simulink library "DAMA_lib"  (Simulink 6.6)
undefined symbols (not defined in the file or in its folder): aa2rot, D, DiscIntNeverNeededParam, DRprogressbar, epsilon, Kd, Ko, Kp, manip, manipulator, path_des, Q, q0, q_d0, rho, robot, show_3D, StartTime, subs, Ts, VR_handle, vrmfunc
libraries: DAMA_lib x7, vrlib x1, simulink x1
(part 1 of 4)
settings Model: Creator=dario  LastModifiedBy=mofo  ExtModeAutoUpdateStatusClock=off

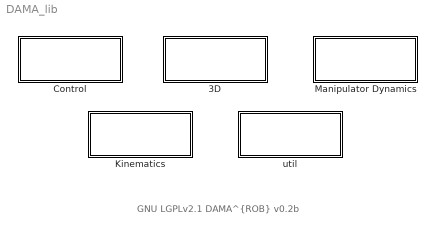
== system DAMA_lib ==
  note: GNU LGPLv2.1 DAMA^{ROB} v0.2b
  3D : Subsystem
  Control : Subsystem
  Kinematics : Subsystem
  Manipulator Dynamics : Subsystem
  util : Subsystem

== system DAMA_lib/3D ==
  note: GNU LGPLv2.1 DAMA^{ROB} v0.2b
  3Dmodel : Subsystem  mask(3D model){sel_obj_nam=Manipulator Name, robot=manipulator, wrlfile=manipVR_base.wrl, SampleTime=0.1, show_ax=off, show_3D_param=off, CaptureFileFormat=png, CaptureFileName='%f_shot_%n.png', Record3D=off, Record3DFileName='%f_anim_%n.wrl', Record2D=off, Record2DCompressMethod=none, Record2DFPS=15, Record2DFileName='%f_anim_%n.avi', Wireframe=off, Viewpoint=STD, RecordMode=scheduled, RecordInterval=[0 10]}
      mask prompts: sel_obj_nam "Input Method"; robot "Manipulator Name"; wrlfile "WRL file name"; SampleTime "3D Sample Time"; show_ax "enable "show axes" input"; show_3D_param "show VRML parameters"; CaptureFileFormat "screenshot file format"; CaptureFileName "screenshot file name (string)"; Record3D "RecordWRL"; Record3DFileName "WRL file name (string)"; Record2D "Record AVI"; Record2DCompressMethod "AVI Compression"; Record2DFPS "AVI FPS"; Record2DFileName "AVI file name (string)"; RecordInterval "Record Interval"
      mask help:
      | Display the 3D model associated with a manipulator.
      |
      | Block Inputs:
      | 1st: signal with joint positions
      | 2nd (if enabled): logical input, if true show frame-axes in 3D animation.
      |
      | Copyright (C) 2009, by Carmine Dario Bellicoso and Marco Caputano.
      | This file is part of DAMA^{ROB} v.???
      | relased under GNU license LGPLv2.1
      mask init:
      | %% SOME INIT
      | mainblock = gcb;
      | blocks = get(gcbh,'Blocks');
      | load_system('DAMA_lib');
      | VR_handle = get_param([gcb,'/VR'],'Handle');
      | % StartTime = str2num(get_param(gcs,'StartTime'));
      | 
      | if strcmp(get_param(gcs,'SimulationStatus'),'stopped')  % operate inside the block only simulation is not running
      |     %% there's something inside the block, delete everything but the inport and VR!
      |     if length(blocks) >= 2
      |         lin = get_param(mainblock,'lines');     % delete lines
      |         if ~isempty(lin)
      |             delete(lin.Handle);
      |         end
      |         for i = 2:1:length(blocks)              % delete blocks
      |             if strcmp(blocks{i},'VR') ~= 1
      |                 delete_block([mainblock,'/',blocks{i}])
      |             end
      |         end
      |         set_param(mainblock,'MaskDisplay', 'disp(''select manipulator'')' );    % change mask aspect
      |         orig_pos = get_param(mainblock,'Position');
      |         new_pos = orig_pos([1,2,1,2]) + [ 0 0 170 65];
      |         set_param(mainblock,'Position', new_pos);
      |     end
      | 
      | 
      |     %% extract information from input data (oject name / WRL file)
      |     if strcmp(sel_obj_nam,'Manipulator Name')
      |         if isa( robot, 'manipulator') && (robot.DH.r ~= 0)
      |             robot_name = robot.name;
      |             DH = robot.DH.table;
      |             r = size(DH)*[1;0];
      |             wrlfile = [robot_name,'VR_base.wrl'];
      |             imagefile = [robot_name,'_3D.png'];
      |         else
      |             return
      |         end
      |     else
      |         if strcmp(sel_obj_nam,'WRL file name')           % WRL file
      |             if exist(wrlfile,'file')
      |                 robot_name = wrlfile(1:end-11);
      |                 imagefile = [robot_name,'_3D.png'];
      |                 f = fopen(wrlfile,'r');
      |                 DH5 = fgetl(f);  %#ok<NASGU>
      |                 DH5 = fgetl(f);
      |                 DH5 = DH5(11:end);
      |                 fclose(f);
      |                 DH5n = eval(DH5);
      |                 r = length(DH5n);
      |                 DH(:,5) = DH5n;
      |             else
      |                 return
      |             end
      |         end
      |     end
      | 
      |     %% specified manipulator or WRL file exists, let's create the subsystem!
      |     if ~exist(imagefile,'file')
      |         imagefile = 'dama_150.png';
      |     end
      |     png = imread(imagefile);
      |     dimY_png = size(png)*[1; 0; 0];
      |     dimX_png = size(png)*[0; 1; 0];
      |     if dimY_png >= 150
      |         dimY = 150;
      |         dimX = round(dimY * dimX_png/dimY_png);
      |     else
      |         dimY = dimY_png;
      |         dimX = dimX_png;
      |     end
      |     Mask_Disp_string = ['image(imread(''',imagefile,'''))',';port_label(''input'',1,''q'');'];
      |     nodes = '';         % VRML nodes to modify
      |     for i = 1:1:r
      |         if DH(i,5) == 0
      |             nodes = [nodes, 'Z', num2str(i-1) ,'.rotation.4.1.double#' ];  %#ok<AGROW>
      |         else
      |             nodes = [nodes, 'Link',num2str(i),'.translation.3#' ];  %#ok<AGROW>
      |         end
      |     end
      | 
      |     for i = 1:1:r
      |         nodes = [nodes,'Xaxis',num2str(i-1),'.scale#']; %#ok<AGROW>
      |         nodes = [nodes,'Yaxis',num2str(i-1),'.scale#']; %#ok<AGROW>
      |         nodes = [nodes,'Zaxis',num2str(i-1),'.scale#']; %#ok<AGROW>
      |     end
      |     nodes = nodes(1:end-1);
      | 
      |     % add demux and connect input 'q' to it
      |     add_block('built-in/demux', [mainblock,'/demux'],...
      |         'DisplayOption','bar',...
      |         'Position','[90,29,95,211]',...
      |         'ShowName','off',...
      |         'Outputs',num2str(r));
      |     add_line(mainblock,'q/1','demux/1');
      | 
      |     % modify VR sink
      |     set_param([mainblock,'/VR'],...
      |         'Position','[360,69,455,141]',...
      |         'WorldFileName',wrlfile,...
      |         'WorldDescription',['3DAMA manipulator: ',robot_name],...
      |         'AutoView','off',...
      |         'SampleTime',num2str(SampleTime),...
      |         'FieldsWritten',nodes, ...
      |         'FigureProperties', '{''Position'', ''Name'', ''Viewpoint'', ''CameraBound'', ''CameraDirection'', ''CameraPosition'', ''CameraUpVector'', ''ZoomFactor'', ''Antialiasing'', ''Headlight'', ''Lighting'', ''NavPanel'', ''StatusBar'', ''ToolBar'', ''Textures'', ''Transparency'', ''Wireframe'', ''NavZones'', ''NavMode'', ''NavSpeed'', ''Record2DCompressMethod'', ''Record2DCompressQuality'', ''Record2D'', ''Record2DFileName'', ''Record2DFPS'';                [5.0000000000000000e+00   9.7000000000000000e+01   7.8400000000000000e+02   5.3800000000000000e+02], ''scara'', ''_untitled_1'', ''on'', [-1.9898756659875949e-02   1.7901367086524811e-01  -9.8364533503023699e-01], [8.8076866149981403e-01  -7.9236092358681276e+00  -7.2561079645852544e-01], [1.9965352243806467e-03   9.8384528836631602e-01   1.7900967126522893e-01], [1.0000000000000000e+00], ''on'', ''on'', ''on'', ''halfbar'', ''on'', ''on'', ''on'', ''on'', ''off'', ''off'', ''examine'', ''normal'', ''auto'', [7.5000000000000000e+01], ''on'', ''%f_anim2_%n.avi'', [1.0000000000000000e+01]}' );
      | 
      |     % add VR rotation and VR translation blocks, with offset and connections
      |     for i = 1:1:length( DH(:,5) )
      |         position = [200, 50, 270, 80] + [0 50 0 50]*(i-1);
      |         if DH(i,5) == 0
      |             add_block('DAMA_lib/util/rotation', [mainblock,'/rotation',num2str(i)]);
      |             set_param([mainblock,'/rotation',num2str(i)],'Position',position);
      |             add_block('built-in/constant', [mainblock,'/offset',num2str(i)]);
      |             set_param([mainblock,'/offset',num2str(i)],'Value','0');                                         % OFFSET HERE
      |             set_param([mainblock,'/offset',num2str(i)],'Position',position - [65,-18,95,-2]);
      |             add_line(mainblock,['rotation',num2str(i),'/1'], ['VR/',num2str(i)]);
      |             add_line(mainblock,['offset',num2str(i),'/1'],['rotation',num2str(i),'/2']);
      |             add_line(mainblock,['demux/',num2str(i)],['rotation',num2str(i),'/1']);
      |         else
      |             add_block('DAMA_lib/util/translation', [mainblock,'/translation',num2str(i)]);
      |             set_param([mainblock,'/translation',num2str(i)],'Position',position);
      |             add_block('built-in/constant', [mainblock,'/offset',num2str(i)]);
      |             set_param([mainblock,'/offset',num2str(i)],'Value','0.5');                                         % OFFSET HERE
      |             set_param([mainblock,'/offset',num2str(i)],'Position',position - [65,-18,95,-2]);
      |             add_line(mainblock,['translation',num2str(i),'/1'], ['VR/',num2str(i)]);
      |             add_line(mainblock,['offset',num2str(i),'/1'],['translation',num2str(i),'/2']);
      |             add_line(mainblock,['demux/',num2str(i)],['translation',num2str(i),'/1']);
      |         end
      |     end
      | 
      |     % add scale control for axes
      |     add_block('built-in/Product',[mainblock,'/show'],...
      |         'Position',[435,212,475,248]);
      |     add_block('built-in/Constant',[mainblock,'/scale'],...
      |         'Value','[1,1,1]',...
      |         'Position','[370,232,410,248]');
      |     add_line(mainblock,'scale/1','show/2');
      |     for i=r+1:1:r+(3*r)
      |         add_line(mainblock,'show/1',['VR/',num2str(i)]);
      |     end
      | 
      |     % inport 2 or constant '1'
      |     if strcmp(get_param(mainblock,'show_ax'),'on')
      |         add_block('built-in/Inport',[mainblock,'/axes_en'],...
      |             'Position','[375,203,405,217]');
      |         Mask_Disp_string = [Mask_Disp_string ,';port_label(''input'',2,''axes'');'];
      |     else
      |         add_block('built-in/Constant',[mainblock,'/axes_en'],...
      |             'Value','1',...
      |             'Position','[375,203,405,217]');
      |     end
      |     add_line(mainblock,'axes_en/1','show/1');
      | 
      |     % change mask aspect
      |     set_param(mainblock,'MaskDisplay',Mask_Disp_string);
      |     orig_pos = get_param(mainblock,'Position');
      |     new_pos = orig_pos([1,2,1,2]) + [ 0 0 dimX dimY];
      |     set_param(mainblock,'Position', new_pos);
      | 
      |     % add 'show 3D' block
      |     %     add_block('DAMA_lib/util/show_3D', [mainblock,'/Show_3D'], ...
      |     %         'Position','[375,286,448,316]');
      | 
      |     vrmfunc('FnOpen', VR_handle );
      |     try
      |         wrl_file = get(get_param([mainblock,'/VR'],'Handle'),'WorldFileName');
      |         list_world_corresp = strfind(get(vrworld(vrsfunc('VRT3ListScenes')),'FileName'),wrl_file);
      |         if length(list_world_corresp) == 1
      |             num_world_found = 1;
      |         else
      |             for i=1:length(list_world_corresp)
      |                 if ~isempty(list_world_corresp{i})
      |                     num_world_found = i;
      |                     break
      |                 end
      |             end
      |         end
      |         ls_wrworlds = vrwho;
      | 
      |         w = ls_wrworlds(num_world_found);
      |         f = get(w, 'Figures');
      |     catch
      |         w = vrworld;
      |         f = vrfigure;
      |     end
      | 
      |     if isvalid(w)
      |         if RecordMode == 1
      |             set(w,'RecordMode','manual');
      |         else
      |             set(w,'RecordMode','scheduled');
      |         end
      |         set(w,'RecordInterval', RecordInterval);
      | 
      |         if Record3D == 0
      |             set(w,'Record3D','off');
      |         else
      |             set(w,'Record3D','on');
      |         end
      |         set(w,'Record3DFileName',Record3DFileName);
      |     end
      | 
      |     if isvalid(f)
      |         if CaptureFileFormat == 1
      |             set(f,'CaptureFileFormat','png');
      |         else
      |             set(f,'CaptureFileFormat','tif');
      |         end
      | 
      |         if Record2D == 0
      |             set(f,'Record2D','off');
      |         else
      |             set(f,'Record2D','on');
      |         end
      | 
      |         if Record2DCompressMethod == 1
      |             set(f,'Record2DCompressMethod','none');
      |         else
      |             set(f,'Record2DCompressMethod','auto');
      |         end
      | 
      |         if Wireframe == 0
      |             set(f,'Wireframe','off');
      |         else
      |             set(f,'Wireframe','on');
      |         end
      | 
      |         if Viewpoint == 1
      |             set(f,'Viewpoint','STD');
      |         elseif Viewpoint == 2
      |             set(f,'Viewpoint','XY_plane');
      |         elseif Viewpoint == 3
      |             set(f,'Viewpoint','XY_perspective');
      |         elseif Viewpoint == 4
      |             set(f,'Viewpoint','left view (XZ)');
      |         elseif Viewpoint == 5
      |             set(f,'Viewpoint','right view (-XZ)');
      |         elseif Viewpoint == 6
      |             set(f,'Viewpoint','rear view (-YZ)');
      |         elseif Viewpoint == 7
      |             set(f,'Viewpoint','front view (-YZ)');
      |         end
      | 
      |         set(f,'Record2DFPS',Record2DFPS);
      |         set(f,'CaptureFileName',CaptureFileName);
      |         set(f,'Record2DFileName',Record2DFileName);
      |     end
      | 
      | else
      | 
      |     try
      |         wrl_file = get(get_param([mainblock,'/VR'],'Handle'),'WorldFileName');
      |         list_world_corresp = strfind(get(vrworld(vrsfunc('VRT3ListScenes')),'FileName'),wrl_file);
      |         if length(list_world_corresp) == 1
      |             num_world_found = 1;
      |         else
      |             for i=1:length(list_world_corresp)
      |                 if ~isempty(list_world_corresp{i})
      |                     num_world_found = i;
      |                     break
      |                 end
      |             end
      |         end
      |         ls_wrworlds = vrwho;
      | 
      |         w = ls_wrworlds(num_world_found);
      |         f = get(w, 'Figures');
      |         if isempty(f)
      |             vrmfunc('FnOpen', VR_handle );
      |         end
      |     catch
      |         w = vrworld;
      |         f = vrfigure;
      |     end
      | 
      |     if isvalid(w)
      |         if RecordMode == 1
      |             set(w,'RecordMode','manual');
      |         else
      |             set(w,'RecordMode','scheduled');
      |         end
      |         set(w,'RecordInterval', RecordInterval);
      | 
      |         if Record3D == 0
      |             set(w,'Record3D','off');
      |         else
      |             set(w,'Record3D','on');
      |         end
      |         set(w,'Record3DFileName',Record3DFileName);
      |     end
      | 
      |     if isvalid(f)
      |         if CaptureFileFormat == 1
      |             set(f,'CaptureFileFormat','png');
      |         else
      |             set(f,'CaptureFileFormat','tif');
      |         end
      | 
      |         if Record2D == 0
      |             set(f,'Record2D','off');
      |         else
      |             set(f,'Record2D','on');
      |         end
      | 
      |         if Record2DCompressMethod == 1
      |             set(f,'Record2DCompressMethod','none');
      |         else
      |             set(f,'Record2DCompressMethod','auto');
      |         end
      | 
      |         if Wireframe == 0
      |             set(f,'Wireframe','off');
      |         else
      |             set(f,'Wireframe','on');
      |         end
      | 
      |         if Viewpoint == 1
      |             set(f,'Viewpoint','STD');
      |         elseif Viewpoint == 2
      |             set(f,'Viewpoint','XY_plane');
      |         elseif Viewpoint == 3
      |             set(f,'Viewpoint','XY_perspective');
      |         elseif Viewpoint == 4
      |             set(f,'Viewpoint','left view (XZ)');
      |         elseif Viewpoint == 5
      |             set(f,'Viewpoint','right view (-XZ)');
      |         elseif Viewpoint == 6
      |             set(f,'Viewpoint','rear view (-YZ)');
      |         elseif Viewpoint == 7
      |             set(f,'Viewpoint','front view (-YZ)');
      |         end
      | 
      |         set(f,'Record2DFPS',Record2DFPS);
      |         set(f,'CaptureFileName',CaptureFileName);
      |         set(f,'Record2DFileName',Record2DFileName);
      |     end
      | end
      mask StyleString: popup(Manipulator Name|WRL file name),edit,edit,edit,checkbox,checkbox,popup(png|tif),edit,checkbox,edit,checkbox,popup(none|auto),edit,edit,checkbox,popup(STD|XY_plane|XY_perspective|left view (XZ)|right view (-XZ)|rear view (-YZ)|front view (-YZ)),popup(manual|scheduled),edit
      mask CallbackString:
      | maskStr = get_param(gcb,'MaskValues');
      | Mask_Vis_Cell_Param = get_param(gcb,'MaskVisibilities');
      | 
      | if strcmp(maskStr{1},'Manipulator Name')
      |     Mask_Vis_Cell_Param{2} = 'on';
      |     Mask_Vis_Cell_Param{3} = 'off';
      | else
      |     Mask_Vis_Cell_Param{2} = 'off';
      |     Mask_Vis_Cell_Param{3} = 'on';
      | end
      | 
      | set_param(gcb,'MaskVisibilities', Mask_Vis_Cell_Param);
      | clear maskStr Mask_Vis_Cell_Param|if strcmp(get_param(gcb,'sel_obj_nam'),'Manipulator Name')
      |     manip_name_param = get_param(gcb,'robot');
      |     if exist(manip_name_param,'var') && isa( eval(manip_name_param), 'manipulator')
      |         % do nothing
      |     else
      |         warndlg([manip_name_param,' is not a valid manipulator name.'])
      |     end
      | end
      | clear manip_name_param|if strcmp(get_param(gcb,'sel_obj_nam'),'WRL file name')
      |     wrl_file_name_param = get_param(gcb,'wrlfile');
      |     if exist(wrl_file_name_param,'file')
      |         % do nothing
      |     else
      |         warndlg([wrl_file_name_param,' does''nt exist.'])
      |     end
      | end
      | clear wrl_file_name_param|||maskStr = get_param(gcb,'MaskValues');
      | Mask_Vis_Cell_Param = get_param(gcb,'MaskVisibilities');
      | 
      | if strcmp(maskStr{6},'on')
      |     for i_mask_par=7:18
      |         Mask_Vis_Cell_Param{i_mask_par} = 'on';
      |     end
      | else
      |     for i_mask_par=7:18
      |         Mask_Vis_Cell_Param{i_mask_par} = 'off';
      |     end
      | end
      | 
      | set_param(gcb,'MaskVisibilities', Mask_Vis_Cell_Param);
      | clear maskStr Mask_Vis_Cell_Param i_mask_par
      | ||||||||||||
      mask Display: disp('select manipulator')

== system DAMA_lib/Control ==
  note: GNU LGPLv2.1 DAMA^{ROB} 0.2b
  Inverse Dynamics : Subsystem  mask(Inverse Dynamics Control){robot=robot, Ts=Ts}
      mask prompts: robot "Robot name ="; Ts "Sampling Time ="
      mask help:
      | Evaluates the control signal given by inverse dynamics compensation for a given manipulator.
      |
      | Copyright (C) 2009, by Carmine Dario Bellicoso and Marco Caputano.
      | This file is part of GNU LGPLv2.1 DAMA^{ROB}
      mask init:
      | n = robot.DH.r; %number of joints
  Manipulator Control : Subsystem  BlockChoice=Robust PD + Inverse Dynamics
      settings: TemplateBlock=self  MemberBlocks=Inverse Dynamics,PD + Inverse Dynamics,Robust PD + Inverse Dynamics
  PD + Inverse Dynamics : Subsystem  mask(Inverse Dynamics with PD control){Kp=Kp, Kd=Kd, robot=robot, Ts=Ts}
      mask prompts: Kp "Proportional Control Gain Matrix="; Kd "Derivative Control Gain Matrix ="; robot "Robot name ="; Ts "Sampling Time ="
      mask help:
      | Evaluates the control signal given by inverse dynamics compensation with a PD controller action for a given manipulator
      |
      | Copyright (C) 2009, by Carmine Dario Bellicoso and Marco Caputano.
      | This file is part of GNU LGPLv2.1 DAMA^{ROB}
      mask init:
      | n = robot.DH.r; %number of joints
  Robust PD + Inverse Dynamics : Subsystem  mask(Robust Control){Kp=Kp, Kd=Kd, Q=Q, D=D, epsilon=epsilon, rho=rho, robot=robot, Ts=Ts}
      mask prompts: Kp "Proportional Control Gain Matrix="; Kd "Derivative Control Gain Matrix ="; Q "Q matrix ="; D "D matrix ="; epsilon "epsilon (chattering) ="; rho "rho gain ="; robot "Robot name ="; Ts "Sampling Time ="
      mask help:
      | Evaluates the control signal given by a robust control for a given manipolator.
      |
      | Copyright (C) 2009, by Carmine Dario Bellicoso and Marco Caputano.
      | This file is part of GNU LGPLv2.1 DAMA^{ROB}
      mask init:
      | n = robot.DH.r; %number of joints

== system DAMA_lib/Kinematics ==
  note: GNU LGPLv2.1 DAMA^{ROB} 0.2b
  Change Frame : Subsystem  mask(Change Frame){manip=manip, inframe=0, outframe=0}
      mask prompts: manip "Manipulator Name:"; inframe "input frame:"; outframe "output frame:"
      mask help:
      | Computes the coordinates of a vector in different frames
      | input:  u  -  input vector
      | output: v -  coordinates of u in new frame
      |
      | note: insert in input/output frame the number of desidered frame.
      | allowed values: (n = number of links)
      |   1..n  = joint frame
      |    -1   = base frame
      |   n+1 =  end-effector frame
      |
      | Copyright (C) 2009
      |  by Carmine Dario Bellicoso and Marco Caputano.
      | This file is part of GNU LGPLv2.1 DAMA^{ROB}
      mask init:
      | % some init
      | thisblock = gcb;
      | if ~isempty(manip) && ~isempty(inframe) && ~isempty(outframe) % some check
      |     if ~isnumeric(inframe) || ~isnumeric(outframe) || inframe < -1 || outframe > manip.DH.r + 1;
      |         set_param(thisblock,'MaskDisplay', 'color(''black'');disp(''Invalid'');' );
      |         T = zeros(4,4);
      |         return
      |     end
      | 
      |     r = manip.DH.r;
      |     Atmp = cell(1,r+2);
      |     T = eye(4);
      |     Atmp{1} = manip.kin.T.Tb0;
      |     Atmp{r+2} = manip.kin.T.Tne;
      |     for i = 1:r
      |         Atmp{i+1} = manip.kin.A.A{i};
      |     end
      | 
      | 
      |     % Toi, o < i
      |     if outframe < inframe
      |         for i = outframe+2:inframe+1
      |             T = T * Atmp{i};
      |         end
      |     elseif inframe < outframe
      |         for i = inframe+2:outframe+1
      |             T = T * Atmp{i};
      |         end
      |         T = inv(T);
      |     end
      |     
      |     % mask: prepare string
      |     if outframe == r+1                    % outframe
      |         dispout = 'e';
      |     elseif outframe >= 0
      |         dispout = num2str(outframe);
      |     elseif outframe == -1
      |         dispout = 'b';
      |     else
      |         dispout='?';
      |     end
      | 
      |     if inframe == r+1                     % inframe
      |         dispin = 'e';
      |     elseif inframe >= 0
      |         dispin = num2str(inframe);
      |     elseif inframe == -1
      |         dispin = 'b';
      |     else
      |         dispin ='?';
      |     end
      |     % mask: update
      |     set_param(gcb,'MaskDisplay', ['color(''black'');disp(''T',dispout,dispin,''');'] );   
      | end
      mask CallbackString:
      | thisblock = gcb;
      | manip_name = get_param(thisblock,'manip');
      | if exist(manip_name,'var') && isa( eval(manip_name), 'manipulator')
      |     if eval([manip_name,'.evaluated.Direct_Kinematics']) == 0
      |         eval([manip_name,'.Direct_Kinematics;']);
      |     end
      | else
      |     warndlg([manip_name,' is not a valid manipulator name.']);
      |     set_param(gcb,'MaskDisplay', 'color(''black'');disp(''Invalid'');' );
      | end
      | clear thisblock manip_name|thisblock = gcb;
      | manip_name = get_param(thisblock,'manip');
      | infr = get_param(thisblock,'inframe');
      | if exist(manip_name,'var') && isa( eval(manip_name), 'manipulator')
      |     try
      |         infrn = eval(infr);
      |         manip_obj = eval(manip_name);
      |         if infrn>=-1 && infrn <= manip_obj.DH.r + 1
      |         else
      |             warndlg('Invalid Input Frame.');
      |             set_param(thisblock,'MaskDisplay', 'color(''black'');disp(''Invalid'');' );
      |         end
      |     catch
      |         warndlg('Invalid Input Frame.');
      |         set_param(thisblock,'MaskDisplay', 'color(''black'');disp(''Invalid'');' );
      |     end
      | end
      | clear thisblock manip_name infr infrn manip_obj|thisblock = gcb;
      | manip_name = get_param(thisblock,'manip');
      | infr = get_param(thisblock,'outframe');
      | if exist(manip_name,'var') && isa( eval(manip_name), 'manipulator')
      |     try
      |         infrn = eval(infr);
      |         manip_obj = eval(manip_name);
      |         if infrn>=-1 && infrn <= manip_obj.DH.r + 1
      |         else
      |             warndlg('Invalid Output Frame.');
      |             set_param(thisblock,'MaskDisplay', 'color(''black'');disp(''Invalid'');' );
      |         end
      |     catch
      |         warndlg('Invalid Output Frame.');
      |         set_param(thisblock,'MaskDisplay', 'color(''black'');disp(''Invalid'');' );
      |     end
      | end
      | clear thisblock manip_name infr infrn manip_obj
      mask Display: color('black');disp('Invalid');
  Direct Kinematics : Subsystem  mask(Direct Kinematics){manip=manipulator}
      mask prompts: manip "Manipulator Name:"
      mask help:
      | Computes direct kinematics of a manipulator.
      | input:  q  -  variable joints
      | output: n s a  -  coordinates of end effector frame unit vectors, expressed in base frame.
      |               p    -  horigin of end effector frame unit vectors, expressed in base frame.
      |
      | Copyright (C) 2009, by Carmine Dario Bellicoso and Marco Caputano.
      | This file is part of GNU LGPLv2.1 DAMA^{ROB}
      mask init:
      | n = manip.DH.r; %number of joints
      mask CallbackString:
      | thisblock = gcb;
      | manip_name = get_param(thisblock,'manip');
      | if exist(manip_name,'var') && isa( eval(manip_name), 'manipulator')
      |     if eval([manip_name,'.evaluated.Direct_Kinematics']) == 0
      |         eval([manip_name,'.Direct_Kinematics;']);
      |     end
      |     set_param(gcb,'MaskDisplay', ['color(''black'');disp(''',manip_name,'\nkine(q)'');'] );
      | else
      |     warndlg([manip_name,' is not a valid manipulator name.']);
      |     set_param(gcb,'MaskDisplay', 'color(''black'');disp(''invalid\nmanipulator'');' );
      | end
      | clear thisblock manip_name
      mask Display: color('black');disp('invalid\nmanipulator');
  Transpose Jacobian Inverse Kinematics : Subsystem  mask(Transpose Jacobian Inverse Kinematics){manip=manipulator, Kp=Kp, Ko=Ko, q0=q0, Ts=0.01}
      mask prompts: manip "manipulator"; Kp "Kp [3x3]"; Ko "Ko [3x3]"; q0 "Initial joints position [rx1]"; Ts "Sample Time"
      mask help: Computes the inverse kinematics of a trajectory in operational space (position only) for a given manipulator (variable stored in robot name).
      mask CallbackString:
      | thisblock = gcb;
      | manip_name = get_param(thisblock,'manip');
      | if exist(manip_name,'var') && isa( eval(manip_name), 'manipulator')
      |     if eval([manip_name,'.evaluated.Direct_Kinematics']) == 0
      |         eval([manip_name,'.Direct_Kinematics;']);
      |     end
      |     set_param(gcb,'MaskDisplay', ['color(''black'');disp(''',manip_name,'\nJ'''' CLIK'');'] );
      | else
      |     warndlg([manip_name,' is not a valid manipulator name.']);
      |     set_param(gcb,'MaskDisplay', 'color(''black'');disp(''invalid\nmanipulator'');' );
      | end
      | clear thisblock manip_name||||
      mask Display: color('black');disp('invalid\nmanipulator');
  trajectory : Subsystem  mask(Trajectory){path_des=path_des}
      mask prompts: path_des "trajectory"
      mask help:
      | Import a trajectory from workspace,
      | created with trajectory.m function.
      |
      | Copyright (C) 2009
      |  by Carmine Dario Bellicoso and Marco Caputano.
      | This file is part of GNU LGPLv2.1 DAMA^{ROB}
      mask Display: color('black')

== system DAMA_lib/Manipulator Dynamics ==
  note: GNU LGPLv2.1 DAMA^{ROB} v.0.2b
  Inertial Load : Subsystem  mask(Load){m=0, Ixx=0, Iyy=0, Izz=0, Ixy=0, Iyz=0, Ixz=0}
      mask prompts: m "Load mass"; Ixy "Ixy ( = Iyx)"; Iyz "Iyz ( = Izy)"; Ixz "Ixz ( = Izx)"
      mask help:
      | Defines the inertia matrix of a load
      | of mass m and inertia tensor I.
      |
      | Copyright (C) 2009,
      | by Carmine Dario Bellicoso and Marco Caputano.
      | This file is part of GNU LGPLv2.1 DAMA^{ROB}
      mask Display: color('black');disp('Inertial Load')
  Manipulator Dynamics : Subsystem  mask(Robot Direct Dynamics){robot=manipulator, q0=q0, qd0=q_d0, fast_enable=on, g_enable=on, Fv_enable=on, lim_enable=off, K_eq=400, b_eq=200}
      mask prompts: robot "Manipulator Name"; q0 "q(0)  - Joint initial positions"; qd0 "q'(0) - Joint initial velocities"; fast_enable "enable fast 2nd order derivative (fast)"; g_enable "enable gravity"; Fv_enable "enable viscous friction"; lim_enable "enable mechanical limits"; K_eq "equivalent stiffness (scalar)"; b_eq "equivalent damping (scalar)"
      mask help:
      | Evaluates joint accelerations, velocities and positions from generalized
      | forces applied to joints (tau) and the generalized forces applied to the
      | end-effector.
      |
      | note:
      | The "enable fast 2nd order derivative" parameter is enabled in default
      | settings, so q_dd are evaluated with 1 simulation step-time delay.
      | If you don't know what that mean, you are strongly encouraged to not
      | change this option.
      | If you intentionally disable this option, you have to know that the block
      | will involve an algebraic loop.
      |
      | Copyright (C) 2009, by Carmine Dario Bellicoso and Marco Caputano.
      | This file is part of GNU LGPLv2.1 DAMA^{ROB}
      mask init:
      | mainblock = gcb;
      | try
      |     n = robot.DH.r;
      |     up_lim = double(robot.DH.table(:,7));
      |     low_lim = double(robot.DH.table(:,6));
      | end
      | load_system('DAMA_lib');
      | if strcmp(get_param(gcs,'SimulationStatus'),'stopped')  % operate inside the block only simulation is not running
      |     % delete 2nd order derivative connections
      |     lines = get_param(mainblock,'Lines');
      |     for i=1:1:length(lines)
      |         if isempty(lines(i).DstBlock) && (strcmp(get(lines(i).Branch(1).DstBlock,'Name'),'q_dd') || strcmp(get(lines(i).Branch(2).DstBlock,'Name'),'q_dd') )
      |             delete(lines(i).Handle);
      |         end
      | 
      |         if isempty(lines(i).DstBlock) && (strcmp(get(lines(i).Branch(1).DstBlock,'Name'),'qdd_mem') || strcmp(get(lines(i).Branch(2).DstBlock,'Name'),'qdd_mem') )
      |             delete(lines(i).Handle);
      |         end
      | 
      |         if isempty(lines(i).DstBlock)
      |             if (strcmp(get(lines(i).Branch(1).DstBlock,'Name'),'qdd_mem') || strcmp(get(lines(i).Branch(2).DstBlock,'Name'),'qdd_mem') )
      |                 delete(lines(i).Handle);
      |             end
      |         else
      |             if strcmp(get(lines(i).DstBlock,'Name'),'qdd_int')
      |                 delete(lines(i).Handle);
      |             end
      |         end
      |     end
      |     try  %#ok<TRYNC>
      |         delete_block([mainblock,'/qdd_mem'])
      |     end
      | 
      |     if fast_enable
      |         % FAST (approx 2nd derivative)
      |         add_block('built-in/memory', [mainblock,'/qdd_mem'],...
      |             'Position', [965   137   990   163]);
      | 
      |         add_line(mainblock, 'invB_tau(xi, q)/1', 'qdd_int/1', 'autorouting','on');
      |         add_line(mainblock, 'invB_tau(xi, q)/1', 'qdd_mem/1', 'autorouting','on');
      | 
      |         add_line(mainblock, 'qdd_mem/1', 'qdd_goto/1', 'autorouting','on');
      |         add_line(mainblock, 'qdd_mem/1', 'q_dd/1', 'autorouting','on');
      |     else
      |         % SLOW (exact 2nd derivative)
      |         add_line(mainblock, 'invB_tau(xi, q)/1', 'qdd_int/1', 'autorouting','on');
      |         add_line(mainblock, 'invB_tau(xi, q)/1', 'qdd_goto/1', 'autorouting','on');
      |         add_line(mainblock, 'invB_tau(xi, q)/1', 'q_dd/1', 'autorouting','on');
      |     end
      | end
      mask CallbackString:
      | thisblock = gcb;
      | manip_name = get_param(thisblock,'robot');
      | if exist(manip_name,'var') && isa( eval(manip_name), 'manipulator')
      |     if eval([manip_name,'.dyndata']) == 1
      |         if eval([manip_name,'.evaluated.Direct_Dynamics']) == 0
      |             if eval([manip_name,'.evaluated.Direct_Kinematics']) == 0
      |                 eval([manip_name,'.Direct_Kinematics;']);
      |             end
      |             eval([manip_name,'.Direct_Dynamics;']);
      |         end
      |         set_param(gcb,'MaskDisplay', ['color(''black'');disp(''',manip_name,'\n\n\n'');'] );
      |     else
      |         set_param(gcb,'MaskDisplay', ['color(''black'');disp(''',manip_name,'\n\n\nmissing dynamic data'');'] );
      |     end
      | else
      |     warndlg([manip_name,' is not a valid manipulator name.']);
      |     set_param(gcb,'MaskDisplay', 'color(''black'');disp(''Invalid\n\n\n'');' );
      | end
      | clear thisblock manip_name||||||maskStr = get_param(gcb,'MaskValues');
      | if strcmp(maskStr{7},'on')
      |     set_param(gcb,'MaskVisibilities',{'on';'on';'on';'on';'on';'on';'on';'on';'on'});
      | else
      |     set_param(gcb,'MaskVisibilities',{'on';'on';'on';'on';'on';'on';'on';'off';'off'});
      | end||
      mask Display: color('black');disp('Invalid\n\n\n');
  wires:
  Inertial Load/1(Load Inertia Matrix) -> Manipulator Dynamics/2(load inertia)

== system DAMA_lib/util ==
  note: VRML INTERFACE
  note: DYNAMICS
  note: GNU LGPLv2.1 DAMA^{ROB} v0.2b
  note: MISC
  B(q)*q_dd : Subsystem  mask(Inertial Forces){robot=robot}
      mask prompts: robot "Manipulator Name:"
      mask help: Evaluates inertial generalized forces acting on manipulator joints.
      mask init:
      | n = robot.DH.r;
  Progress Bar : Subsystem  mask(Progress Bar){}
      mask help: Show a progressbar during simulation.
      mask init:
      | t_f = eval(get_param(get_param(gcb,'Parent'),'StopTime'));
      | h = waitbar(0,'Simulating system...   ');
      | set(h,'Visible','off');
      | Ts = t_f / 100;
      mask Display: image(imread('progress.png'));
  n(q,q_d) : Subsystem  mask(NonLinear Forces){robot=robot}
      mask prompts: robot "Manipulator Name:"
      mask help:
      | Evaluates non linear generalized forces acting on manipulator joints due to:
      |  -  gravitational field
      |  -  centripetal-Coriolis accelerations
      |  -  viscous friction
      mask init:
      | n = robot.DH.r;
  rotation : Subsystem
      mask Type: VRML rotation
      mask Description:
      | Implement a Z-axis VRML rotation vector
      | 1st input: rotation angle
      | 2nd input: rotation offset
  show_3D : Subsystem
      mask Type: Show 3D window
      mask Description: Prevent 3D window closing
      mask Display: disp('show 3D')
  translation : Subsystem
      mask Type: VRML translation
      mask Description:
      | Implement a Z-axis VRML translation vector
      | 1st input: translation value
      | 2nd input: translation offset

== system DAMA_lib/3D/3Dmodel ==
  q : Inport
  VR : vrlib/VR Sink  SampleTime=0.1  ViewEnable=on  RemoteChange=off  RemoteView=on  WorldDescription=3DAMA manipulator: manip3  AutoView=off  FigureProperties="{'Position', 'Name', 'Viewpoint', 'CameraBound', 'CameraDirection', 'CameraPosition', 'CameraUpVector', 'ZoomFactor', 'Antialiasing', 'Headlight', 'Lighting', 'NavPanel', 'StatusBar', 'ToolBar', 'Textures', 'Transparency', 'Wireframe', 'NavZones', 'NavMode', 'NavSpeed', 'Record2DCompressMethod', 'Record2DCompressQuality', 'Record2D', 'Record2DFileName', 'Record2DFPS';                [5.0000000000000000e+00   9.7000000000000000e+01   7.8400000000000000e+02   5.3800000000000000e+02], 'scara', '_untitled_1', 'on', [-1.9898756659875949e-02   1.7901367086524811e-01  -9.8364533503023699e-01], [8.8076866149981403e-01  -7.9236092358681276e+00  -7.2561079645852544e-01], [1.9965352243806467e-03   9.8384528836631602e-01   1.7900967126522893e-01], [1.0000000000000000e+00], 'on', 'on', 'on', 'halfbar', 'on', 'on', 'on', 'on', 'off', 'off', 'examine', 'normal', 'auto', [7.5000000000000000e+01], 'on', '%f_anim2_%n.avi', [1.0000000000000000e+01]}"

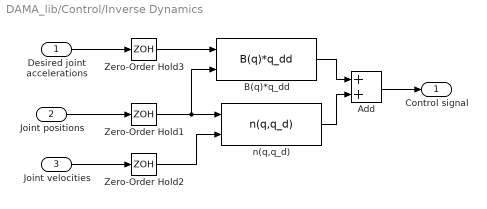
== system DAMA_lib/Control/Inverse Dynamics ==
  Desired joint accelerations : Inport
  Joint positions : Inport  Port=2
  Joint velocities : Inport  Port=3
  Add : Sum  OutScaling=2^-10
  B(q)*q_dd : DAMA_lib/util/B(q)*q_dd  SystemSampleTime=-1  robot=robot
  Zero-Order Hold1 : ZeroOrderHold  SampleTime=Ts
  Zero-Order Hold2 : ZeroOrderHold  SampleTime=Ts
  Zero-Order Hold3 : ZeroOrderHold  SampleTime=Ts
  n(q,q_d) : DAMA_lib/util/n(q,q_d)  SystemSampleTime=-1  robot=robot
  Control signal : Outport
  wires:
  Desired joint accelerations/1 -> Zero-Order Hold3/1
  Add/1 -> Control signal/1
  n(q,q_d)/1 -> Add/2
  B(q)*q_dd/1 -> Add/1
  Joint positions/1 -> Zero-Order Hold1/1
  Joint velocities/1 -> Zero-Order Hold2/1
  Zero-Order Hold3/1 -> B(q)*q_dd/1
  Zero-Order Hold1/1 -> B(q)*q_dd/2, n(q,q_d)/1
  Zero-Order Hold2/1 -> n(q,q_d)/2

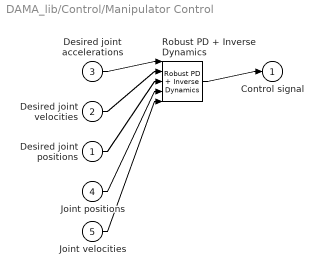
== system DAMA_lib/Control/Manipulator Control ==
  Desired joint positions : Inport
  Desired joint velocities : Inport  Port=2
  Desired joint accelerations : Inport  Port=3
  Joint positions : Inport  Port=4
  Joint velocities : Inport  Port=5
  Robust PD + Inverse Dynamics : DAMA_lib/Control/Robust PD + Inverse Dynamics  SystemSampleTime=-1  Kp=Kp  Kd=Kd  Q=Q  D=D  epsilon=epsilon  rho=rho  robot=robot  Ts=Ts
  Control signal : Outport
  wires:
  Desired joint accelerations/1 -> Robust PD + Inverse Dynamics/1
  Desired joint velocities/1 -> Robust PD + Inverse Dynamics/2
  Desired joint positions/1 -> Robust PD + Inverse Dynamics/3
  Joint positions/1 -> Robust PD + Inverse Dynamics/4
  Joint velocities/1 -> Robust PD + Inverse Dynamics/5
  Robust PD + Inverse Dynamics/1 -> Control signal/1

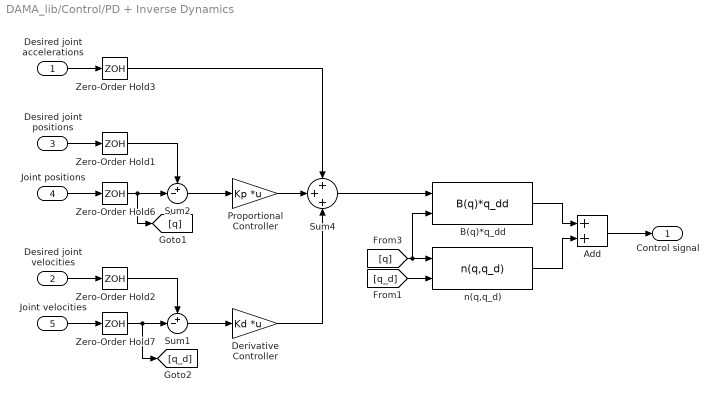
== system DAMA_lib/Control/PD + Inverse Dynamics ==
  Desired joint accelerations : Inport
  Desired joint velocities : Inport  Port=2
  Desired joint positions : Inport  Port=3
  Joint positions : Inport  Port=4
  Joint velocities : Inport  Port=5
  Add : Sum  OutScaling=2^-10
  B(q)*q_dd : DAMA_lib/util/B(q)*q_dd  SystemSampleTime=-1  robot=robot
  Derivative Controller : Gain  Gain=Kd  Multiplication=Matrix(K*u)
  Proportional Controller : Gain  Gain=Kp  Multiplication=Matrix(K*u)
  Sum1 : Sum  Inputs=+-|
  Sum2 : Sum  Inputs=+-|
  Sum4 : Sum  Inputs=+++
  Zero-Order Hold{1..3,6..7} (5 alike) : ZeroOrderHold  SampleTime=Ts
  n(q,q_d) : DAMA_lib/util/n(q,q_d)  SystemSampleTime=-1  robot=robot
  Control signal : Outport
  wires:
  Desired joint accelerations/1 -> Zero-Order Hold3/1
  Add/1 -> Control signal/1
  n(q,q_d)/1 -> Add/2
  B(q)*q_dd/1 -> Add/1
  Joint positions/1 -> Zero-Order Hold6/1
  Desired joint positions/1 -> Zero-Order Hold1/1
  Joint velocities/1 -> Zero-Order Hold7/1
  Desired joint velocities/1 -> Zero-Order Hold2/1
  Zero-Order Hold1/1 -> Sum2/1
  Sum1/1 -> Derivative Controller/1
  Sum2/1 -> Proportional Controller/1
  Zero-Order Hold2/1 -> Sum1/1
  Zero-Order Hold7/1 -> Sum1/2, [q_d]
  Zero-Order Hold6/1 -> Sum2/2, [q]
  [q] -> n(q,q_d)/1, B(q)*q_dd/2
  [q_d] -> n(q,q_d)/2
  Proportional Controller/1 -> Sum4/2
  Derivative Controller/1 -> Sum4/3
  Sum4/1 -> B(q)*q_dd/1
  Zero-Order Hold3/1 -> Sum4/1

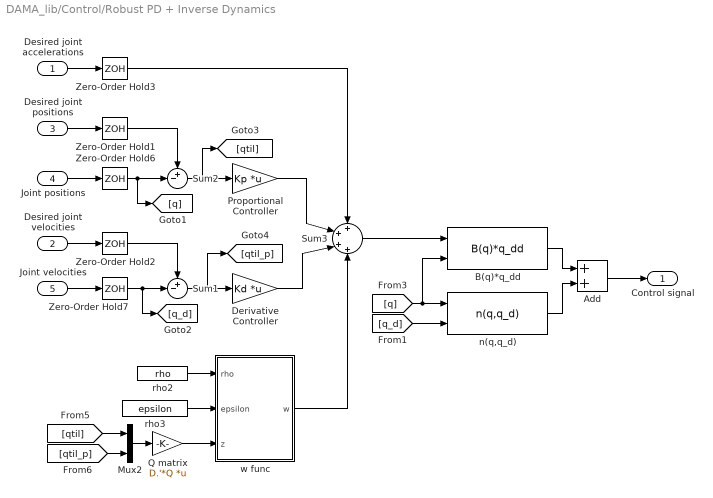
== system DAMA_lib/Control/Robust PD + Inverse Dynamics ==
  Desired joint accelerations : Inport
  Desired joint velocities : Inport  Port=2
  Desired joint positions : Inport  Port=3
  Joint positions : Inport  Port=4
  Joint velocities : Inport  Port=5
  Add : Sum  OutScaling=2^-10
  B(q)*q_dd : DAMA_lib/util/B(q)*q_dd  SystemSampleTime=-1  robot=robot
  Derivative Controller : Gain  Gain=Kd  Multiplication=Matrix(K*u)
  Mux2 : Mux  Inputs=2
  Proportional Controller : Gain  Gain=Kp  Multiplication=Matrix(K*u)
  Q matrix : Gain  Gain=D.'*Q  Multiplication=Matrix(K*u) (u vector)
  Sum1 : Sum  Inputs=+-|
  Sum2 : Sum  Inputs=+-|
  Sum3 : Sum  Inputs=++++
  Zero-Order Hold{1..3,6..7} (5 alike) : ZeroOrderHold  SampleTime=Ts
  n(q,q_d) : DAMA_lib/util/n(q,q_d)  SystemSampleTime=-1  robot=robot
  rho2 : Constant  Value=rho
  rho3 : Constant  Value=epsilon
  w func : Subsystem
  Control signal : Outport
  wires:
  Desired joint accelerations/1 -> Zero-Order Hold3/1
  Add/1 -> Control signal/1
  Joint positions/1 -> Zero-Order Hold6/1
  Desired joint positions/1 -> Zero-Order Hold1/1
  Joint velocities/1 -> Zero-Order Hold7/1
  Desired joint velocities/1 -> Zero-Order Hold2/1
  Zero-Order Hold1/1 -> Sum2/1
  Sum1/1 -> Derivative Controller/1, [qtil_p]
  Sum2/1 -> Proportional Controller/1, [qtil]
  Zero-Order Hold2/1 -> Sum1/1
  Zero-Order Hold7/1 -> Sum1/2, [q_d]
  Zero-Order Hold6/1 -> Sum2/2, [q]
  [q] -> B(q)*q_dd/2, n(q,q_d)/1
  [q_d] -> n(q,q_d)/2
  Zero-Order Hold3/1 -> Sum3/1
  Proportional Controller/1 -> Sum3/2
  Derivative Controller/1 -> Sum3/3
  B(q)*q_dd/1 -> Add/1
  Sum3/1 -> B(q)*q_dd/1
  n(q,q_d)/1 -> Add/2
  Mux2/1 -> Q matrix/1
  [qtil] -> Mux2/1
  [qtil_p] -> Mux2/2
  rho2/1 -> w func/1(rho)
  Q matrix/1 -> w func/3(z)
  rho3/1 -> w func/2(epsilon)
  w func/1(w) -> Sum3/4

== system DAMA_lib/Kinematics/Change Frame ==
  q : Inport
  u : Inport  Port=2
  Constant6 : Constant
  Mux1 : Mux  Inputs=2
  Product : Product  Multiplication=Matrix(*)  RndMeth=Zero
  T : MATLABFcn  MATLABFcn=subs(T,manip.jointvar.q,u)  Output1D=off
  v : Outport
  wires:
  T/1 -> Product/1
  Mux1/1 -> Product/2
  Constant6/1 -> Mux1/2
  u/1 -> Mux1/1
  Product/1 -> v/1
  q/1 -> T/1

== system DAMA_lib/Kinematics/Direct Kinematics ==
  q : Inport
  Demux : Demux  Outputs=[3 3 3 3]
  pos norm : MATLABFcn  MATLABFcn=manip.func.nsap(u)
  n : Outport
  s : Outport  Port=2
  a : Outport  Port=3
  p : Outport  Port=4
  wires:
  q/1 -> pos norm/1
  pos norm/1 -> Demux/1
  Demux/1 -> n/1
  Demux/2 -> s/1
  Demux/3 -> a/1
  Demux/4 -> p/1

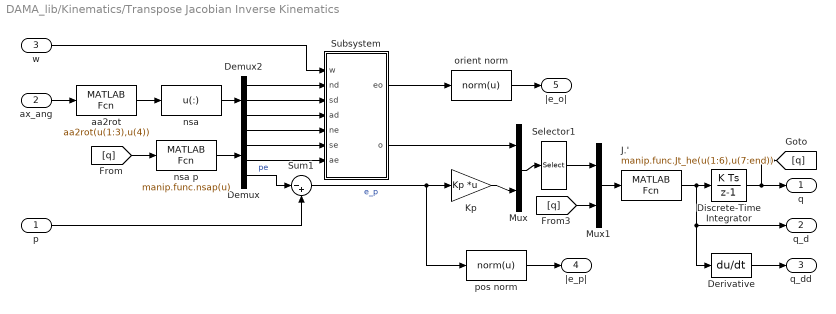
== system DAMA_lib/Kinematics/Transpose Jacobian Inverse Kinematics ==
  p : Inport
  ax_ang : Inport  Port=2  PortDimensions=4
  w : Inport  Port=3  PortDimensions=3
  Demux : Demux  Outputs=[3 3 3 3]
  Demux2 : Demux  Outputs=3
  Derivative : Derivative
  Discrete-Time Integrator : DiscreteIntegrator  InitialCondition=q0  SampleTime=Ts  ICPrevOutput=DiscIntNeverNeededParam  ICPrevScaledInput=DiscIntNeverNeededParam
  J.' : MATLABFcn  MATLABFcn=manip.func.Jt_he(u(1:6),u(7:end))
  Kp : Gain  Gain=Kp  Multiplication=Matrix(K*u) (u vector)
  Mux : Mux  Inputs=2
  Mux1 : Mux  Inputs=2
  Selector1 : Selector  IndexOptions=Index vector (dialog)  Indices=[4:6,1:3]  OutputSizes=1  InputPortWidth=6
  Subsystem : Subsystem
  Sum1 : Sum  Inputs=|-+
  aa2rot : MATLABFcn  MATLABFcn=aa2rot(u(1:3),u(4))  Output1D=off
  nsa : MATLABFcn  MATLABFcn=u(:)
  nsa p : MATLABFcn  MATLABFcn=manip.func.nsap(u)
  orient norm : MATLABFcn  MATLABFcn=norm(u)
  pos norm : MATLABFcn  MATLABFcn=norm(u)
  q : Outport
  q_d : Outport  Port=2
  q_dd : Outport  Port=3
  |e_p| : Outport  Port=4
  |e_o| : Outport  Port=5
  wires:
  Subsystem/2(o) -> Mux/1
  Subsystem/1(eo) -> orient norm/1
  w/1 -> Subsystem/1(w)
  Demux/3 -> Subsystem/7(ae)
  Demux/2 -> Subsystem/6(se)
  Demux/1 -> Subsystem/5(ne)
  Demux2/3 -> Subsystem/4(ad)
  Demux2/2 -> Subsystem/3(sd)
  Demux2/1 -> Subsystem/2(nd)
  nsa/1 -> Demux2/1
  aa2rot/1 -> nsa/1
  Derivative/1 -> q_dd/1
  orient norm/1 -> |e_o|/1
  pos norm/1 -> |e_p|/1
  Sum1/1 -> pos norm/1, Kp/1  "e_p"
  Kp/1 -> Mux/2
  ax_ang/1 -> aa2rot/1
  Demux/4 -> Sum1/1  "pe"
  p/1 -> Sum1/2
  [q] -> nsa p/1
  Mux/1 -> Selector1/1
  Selector1/1 -> Mux1/1
  Mux1/1 -> J.'/1
  [q] -> Mux1/2
  J.'/1 -> Derivative/1, q_d/1, Discrete-Time Integrator/1
  Discrete-Time Integrator/1 -> q/1, [q]
  nsa p/1 -> Demux/1

== system DAMA_lib/Kinematics/trajectory ==
  From Workspace : FromWorkspace  VariableName=path_des.pos  SampleTime=0  OutputAfterFinalValue=Holding final value
  From Workspace1 : FromWorkspace  VariableName=path_des.orient.aa  SampleTime=0  OutputAfterFinalValue=Holding final value
  From Workspace2 : FromWorkspace  VariableName=path_des.w  SampleTime=0  OutputAfterFinalValue=Holding final value
  pos : Outport  OutDataType=fixdt(1,16,0)  OutScaling=[]
  ax_ang : Outport  Port=2  OutDataType=fixdt(1,16,0)  OutScaling=[]
  w : Outport  Port=3  OutDataType=fixdt(1,16,0)  OutScaling=[]
  wires:
  From Workspace2/1 -> w/1
  From Workspace1/1 -> ax_ang/1
  From Workspace/1 -> pos/1

== system DAMA_lib/Manipulator Dynamics/Inertial Load ==
  Tensor : Constant  Value=[m*eye(3) zeros(3,3) ; zeros(3,3) [Ixx -Ixy -Ixz; -Ixy Iyy -Iyz; -Ixz -Iyz Izz]]
  Load Inertia Matrix : Outport
  wires:
  Tensor/1 -> Load Inertia Matrix/1

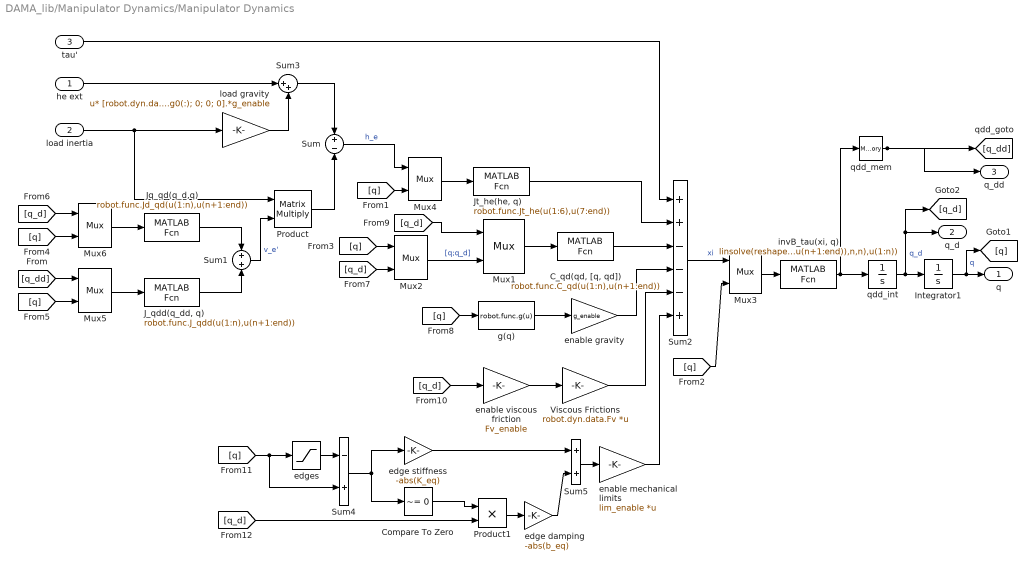
== system DAMA_lib/Manipulator Dynamics/Manipulator Dynamics ==
  he ext : Inport
  load inertia : Inport  Port=2  OutDataType=fixdt(1,16,0)  OutScaling=[]
  tau' : Inport  Port=3  OutDataType=fixdt(1,16,0)  OutScaling=[]
  "C_qd(qd, [q, qd])" : MATLABFcn  MATLABFcn=robot.func.C_qd(u(1:n),u(n+1:end))  OutputDimensions=n
  Compare To Zero : simulink/Logic and Bit Operations/Compare To Zero  SystemSampleTime=-1  relop=~=  LogicOutDataTypeMode=uint8
  Integrator1 : Integrator  InitialCondition=q0  UpperSaturationLimit=[pi/2 pi/4 1 2*pi]  LowerSaturationLimit=[-pi/2 -pi/2 0.25 -2*pi]
  "J_qdd(q_dd, q)" : MATLABFcn  MATLABFcn=robot.func.J_qdd(u(1:n),u(n+1:end))  OutputDimensions=6
  Jq_qd(q_d,q) : MATLABFcn  MATLABFcn=robot.func.Jd_qd(u(1:n),u(n+1:end))  OutputDimensions=6
  "Jt_he(he, q)" : MATLABFcn  MATLABFcn=robot.func.Jt_he(u(1:6),u(7:end))  OutputDimensions=n
  Mux{1..6} (6 alike) : Mux  Inputs=2
      settings: DisplayOption=signals
  Product : Product  Multiplication=Matrix(*)  RndMeth=Zero
  Product1 : Product  RndMeth=Zero
  Sum : Sum  Inputs=+-
  Sum1 : Sum
  Sum2 : Sum  Inputs=++---+
  Sum3 : Sum  Inputs=|++
  Sum4 : Sum  Inputs=-+
  Sum5 : Sum
  Viscous Frictions : Gain  Gain=robot.dyn.data.Fv  Multiplication=Matrix(K*u)
  edge damping : Gain  Gain=-abs(b_eq)
  edge stiffness : Gain  Gain=-abs(K_eq)
  edges : Saturate  UpperLimit=up_lim  LowerLimit=low_lim
  enable gravity : Gain  Gain=g_enable
  enable mechanical limits : Gain  Gain=lim_enable  Multiplication=Matrix(K*u)
  enable viscous friction : Gain  Gain=Fv_enable
  g(q) : MATLABFcn  MATLABFcn=robot.func.g(u)  OutputDimensions=n
  "invB_tau(xi, q)" : MATLABFcn  MATLABFcn=linsolve(reshape(robot.func.B_matrix(u(n+1:end)),n,n),u(1:n))  OutputDimensions=n
  load gravity : Gain  Gain=[robot.dyn.data.g0(:); 0; 0; 0].*g_enable  Multiplication=Matrix(u*K)
  qdd_int : Integrator  InitialCondition=qd0
  qdd_mem : Memory
  q : Outport  OutDataType=fixdt(1,16,0)  OutScaling=[]
  q_d : Outport  Port=2  OutDataType=fixdt(1,16,0)  OutScaling=[]
  q_dd : Outport  Port=3  OutDataType=fixdt(1,16,0)  OutScaling=[]
  wires:
  qdd_mem/1 -> q_dd/1, [q_dd]
  "invB_tau(xi, q)"/1 -> qdd_mem/1, qdd_int/1
  qdd_int/1 -> Integrator1/1, q_d/1, [q_d]  "q_d"
  Integrator1/1 -> q/1, [q]  "q"
  Mux1/1 -> "C_qd(qd, [q, qd])"/1
  Mux2/1 -> Mux1/2  "[q;q_d]"
  "C_qd(qd, [q, qd])"/1 -> Sum2/3
  g(q)/1 -> enable gravity/1
  Mux3/1 -> "invB_tau(xi, q)"/1
  Sum2/1 -> Mux3/1  "xi"
  load inertia/1 -> Product/1, load gravity/1
  Mux5/1 -> "J_qdd(q_dd, q)"/1
  Mux6/1 -> Jq_qd(q_d,q)/1
  Jq_qd(q_d,q)/1 -> Sum1/1
  "J_qdd(q_dd, q)"/1 -> Sum1/2
  Sum1/1 -> Product/2  "v_e'"
  Product/1 -> Sum/2
  Sum/1 -> Mux4/1  "h_e"
  Mux4/1 -> "Jt_he(he, q)"/1
  [q_dd] -> Mux5/1
  [q] -> Mux4/2
  [q] -> Mux2/1
  [q] -> Mux6/2
  [q] -> Mux5/2
  [q_d] -> Mux6/1
  [q_d] -> Mux2/2
  [q] -> g(q)/1
  [q] -> Mux3/2
  tau'/1 -> Sum2/1
  "Jt_he(he, q)"/1 -> Sum2/2
  [q_d] -> Mux1/1
  he ext/1 -> Sum3/1
  Sum3/1 -> Sum/1
  load gravity/1 -> Sum3/2
  enable gravity/1 -> Sum2/4
  enable viscous friction/1 -> Viscous Frictions/1
  [q_d] -> enable viscous friction/1
  Viscous Frictions/1 -> Sum2/5
  edges/1 -> Sum4/1
  Sum4/1 -> Compare To Zero/1, edge stiffness/1
  Compare To Zero/1 -> Product1/1
  Product1/1 -> edge damping/1
  edge damping/1 -> Sum5/2
  [q] -> edges/1, Sum4/2
  [q_d] -> Product1/2
  edge stiffness/1 -> Sum5/1
  Sum5/1 -> enable mechanical limits/1
  enable mechanical limits/1 -> Sum2/6

== system DAMA_lib/util/B(q)*q_dd ==
  q_dd : Inport
  q : Inport  Port=2
  B*q_dd : MATLABFcn  MATLABFcn=robot.func.B_qdd(u(1:n),u(n+1:end))  OutputDimensions=n
  Mux6 : Mux  Inputs=2
      settings: DisplayOption=signals
  inertial_tau : Outport
  wires:
  B*q_dd/1 -> inertial_tau/1
  q/1 -> Mux6/2  "q"
  q_dd/1 -> Mux6/1  "q_dd"
  Mux6/1 -> B*q_dd/1

== system DAMA_lib/util/Progress Bar ==
  Clock : Clock
      settings: Decimation=10000
  End time : Constant  Value=t_f
  Mux1 : Mux
  Progress Bar : MATLABFcn  MATLABFcn=DRprogressbar(u(1),u(2),u(3),u(4))
  Sample time : Constant  Value=Ts
  Stop Simulation : Stop
  bar handle : Constant  Value=h
  wires:
  Sample time/1 -> Mux1/4
  bar handle/1 -> Mux1/3
  End time/1 -> Mux1/2
  Mux1/1 -> Progress Bar/1
  Clock/1 -> Mux1/1
  Progress Bar/1 -> Stop Simulation/1
